simulink model "Arrays2_tmp"  (Simulink 8.3)
settings: Solver=FixedStepDiscrete  StartTime=0.0  StopTime=10000.0  RelTol=1e-3
settings Model: Creator=scaife  LastModifiedBy=bourbouh  CovSFcnEnable=on  ExtModeAutoUpdateStatusClock=off
settings DataIOCC: SignalLoggingName=sigsOut
settings DebuggingCC: SaveWithParameterizedLinksMsg=none  SignalResolutionControl=TryResolveAllWithWarning  SolverPrmCheckMsg=none  MultiTaskDSMMsg=warning  MultiTaskCondExecSysMsg=none  FrameProcessingCompatibilityMsg=error  StateNameClashWarn=none  StrictBusMsg=None
settings HardwareCC: TargetUnknown=on
settings SFSimCC: SimParseCustomCode=off
settings GRTTargetCC: GeneratePreprocessorConditionals=Use local settings

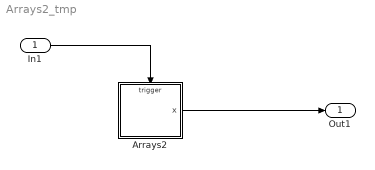
== system Arrays2_tmp ==
  In1 : Inport
  Arrays2 : Stateflow chart  TreatAsAtomicUnit=on
      settings: PermitHierarchicalResolution=ParametersOnly
  Out1 : Outport
  wires:
  In1/1 -> Arrays2/Trigger
  Arrays2/1(x) -> Out1/1

== stateflow chart Arrays2 ==
  state A/
    en:x[1][1]++
    x[2][1]--
  state B/
    en:x[1][2]++
    x[2][2]--
  state C/
    en:x[1][3]++
    x[2][3]--
  (default) -> A
  A -> B : E
  C -> A : E
  B -> C : E
  data: x output double size=[2 3] [0..100] =1
  events: E input RISING_EDGE_EVENT
